simulink subsystem "ESC_Speed_to_PWM_Count"  (R2024b)
settings: Solver=VariableStepAuto  StartTime=0.0  StopTime=10.0  RelTol=1e-3
settings Model: Creator=loq  LastModifiedBy=loq

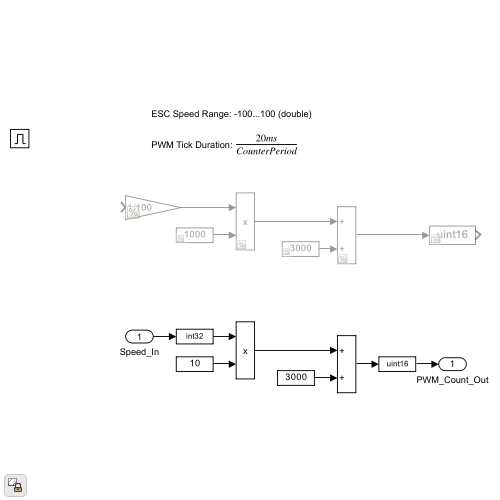
[thumbnail: Simulink's stored preview of the top-level diagram]
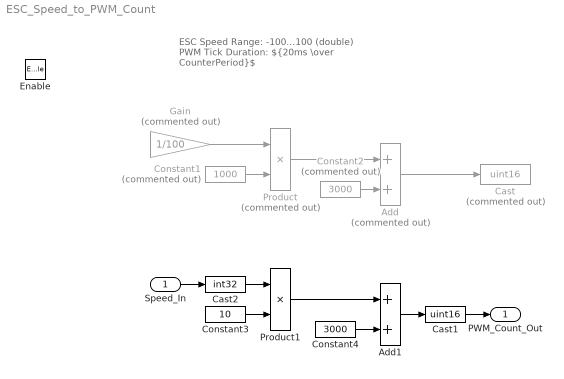
== system ESC_Speed_to_PWM_Count ==
  note: ESC Speed Range: -100...100 (double)
      |
      | PWM Tick Duration: ${20ms \over CounterPeriod}$
  Speed_In : Inport  OutDataTypeStr=int8
  Enable : EnablePort
  Add : Sum  Commented=on
  Add1 : Sum
  Cast : DataTypeConversion  Commented=on  OutDataTypeStr=uint16  SaturateOnIntegerOverflow=off  RndMeth=Floor
  Cast1 : DataTypeConversion  OutDataTypeStr=uint16  SaturateOnIntegerOverflow=off  RndMeth=Floor
  Cast2 : DataTypeConversion  OutDataTypeStr=int32  SaturateOnIntegerOverflow=off  RndMeth=Floor
  Constant1 : Constant  Commented=on  Value=1000
  Constant2 : Constant  Commented=on  Value=3000
  Constant3 : Constant  Value=10  OutDataTypeStr=int32
  Constant4 : Constant  Value=3000  OutDataTypeStr=int32
  Gain : Gain  Commented=on  Gain=1/100
  Product : Product  Commented=on
  Product1 : Product
  PWM_Count_Out : Outport  OutDataTypeStr=uint16  OutputWhenDisabled=reset  InitialOutput=[0]
  wires:
  Constant1/1 -> Product/2
  Constant2/1 -> Add/2
  Add/1 -> Cast/1
  Product/1 -> Add/1
  Gain/1 -> Product/1
  Constant3/1 -> Product1/2
  Constant4/1 -> Add1/2
  Product1/1 -> Add1/1
  Add1/1 -> Cast1/1
  Speed_In/1 -> Cast2/1
  Cast2/1 -> Product1/1
  Cast1/1 -> PWM_Count_Out/1
